simulink model "Impedance"  (R2022b)
settings: Solver=ode113  StartTime=0.0  StopTime=30  RelTol=1e-3
values from neighbouring files (symbols this model uses):
  a_1 = 1    [parameters.m]
  a_2 = 1    [parameters.m]
  kp_1 = 2500    [parameters.m]
  kp_2 = 2500    [parameters.m]
  md_1 = 100    [parameters.m]
  md_2 = 100    [parameters.m]
  xd_1 = 0.75    [parameters.m]
  xd_2 = 0.25    [parameters.m]
settings Model: Creator=eleves  LastModifiedBy=eleves
settings ModelReferenceCC: ModelReferenceMinAlgLoopOccurrences=on

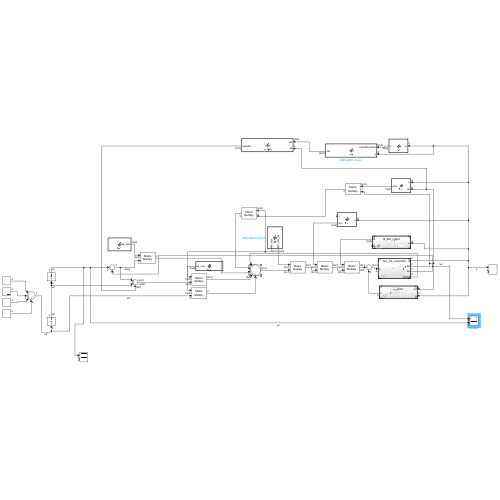
[thumbnail: Simulink's stored preview of the top-level diagram]
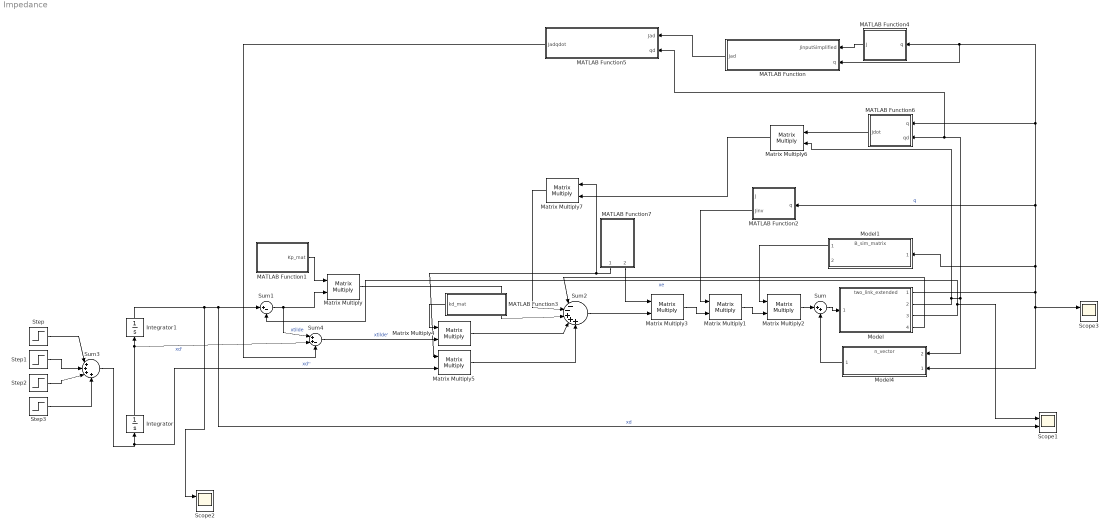
== system Impedance ==
  Integrator : Integrator  InitialCondition=[0;0]
  Integrator1 : Integrator  InitialCondition=[xd_1;xd_2]
  MATLAB Function : MATLAB Function  TreatAsAtomicUnit=on
  MATLAB Function1 : MATLAB Function  TreatAsAtomicUnit=on
  MATLAB Function2 : MATLAB Function  TreatAsAtomicUnit=on
  MATLAB Function3 : MATLAB Function  TreatAsAtomicUnit=on
  MATLAB Function4 : MATLAB Function  TreatAsAtomicUnit=on
  MATLAB Function5 : MATLAB Function  TreatAsAtomicUnit=on
  MATLAB Function6 : MATLAB Function  TreatAsAtomicUnit=on
  MATLAB Function7 : MATLAB Function  TreatAsAtomicUnit=on
  Matrix Multiply{,1..7} (8 alike) : Product  Multiplication=Matrix(*)
  Model : ModelReference  ModelNameDialog=two_link_extended.slx  SimulationMode=Normal  ModelReferenceVersion=1.3
  Model1 : ModelReference  ModelNameDialog=B_sim_matrix.slx  SimulationMode=Normal  ModelReferenceVersion=13.0
  Model4 : ModelReference  ModelNameDialog=n_vector.slx  SimulationMode=Normal  ModelReferenceVersion=1.3
      settings: PortSchema="{\"entries\":[{\"content\":{\"sides\":[{\"content\":{\"connectorIds\":[\"In2\",\"In1\"]},\"type\":\"ConnectorPlacement.EquallySpacedRectSide\",\"uuid\":\"0004a852-6b57-412e-a247-f7a948c02aef\"},{\"content\":{\"connectorIds\":[\"Out1\"],\"side\":\"RIGHT\"},\"type\":\"ConnectorPlacement.EquallySpacedRectSide\",\"uuid\":\"2c6a1f56-b264-4a50-8175-f4e8d5862eda\"},{\"content\":{\"connectorIds\":[],\"side\":\"TOP\"},\"type\":\"ConnectorPlacement.EquallySpacedRectSide\",\"uuid\":\"b3451316-5974-4a81-98c7-74555a3ec881\"}]},\"type\":\"ConnectorPlacement.EquallySpacedConnector\",\"uuid\":\"ac2390f0-df41-4187-a0e3-0c9a5394d303\"}],\"packageUris\":[\"http://schema.mathworks.com/mf0/Connector/R2020b\"],\"version\":\"1.0\"}"
  Scope1 : Scope  NumInputPorts=2
  Scope2 : Scope  NumInputPorts=2
  Scope3 : Scope  NumInputPorts=2
  Step : Step  Time=0  Before=[0.0;0.00]  After=[0.1;0.05]  SampleTime=0
  Step1 : Step  Before=[0.0;0.00]  After=[-0.1;-0.05]  SampleTime=0
  Step2 : Step  Time=5  Before=[0.0;0.00]  After=[-0.1;-0.05]  SampleTime=0
  Step3 : Step  Time=6  Before=[0.0;0.00]  After=[0.1;0.05]  SampleTime=0
  Sum : Sum  Inputs=|++
  Sum1 : Sum  Inputs=|+-
  Sum2 : Sum  Inputs=|--+++
  Sum3 : Sum  Inputs=|++++
  Sum4 : Sum  Inputs=|++-
  wires:
  Sum1/1 -> Sum4/1, Matrix Multiply/2  "xtilde"
  MATLAB Function1/1(Kp_mat) -> Matrix Multiply/1
  Model4/1 -> Sum/2
  Model1/1 -> Matrix Multiply2/1
  Matrix Multiply2/1 -> Sum/1
  Matrix Multiply1/1 -> Matrix Multiply2/2
  MATLAB Function2/2(Jinv) -> Matrix Multiply1/1
  Matrix Multiply3/1 -> Matrix Multiply1/2
  MATLAB Function7/2(Md_mat_inv) -> Matrix Multiply3/1
  Sum2/1 -> Matrix Multiply3/2
  Step/1 -> Sum3/1
  Step1/1 -> Sum3/2
  Step2/1 -> Sum3/3
  Step3/1 -> Sum3/4
  Sum3/1 -> Matrix Multiply5/2, Integrator/1  "xd''"
  Integrator1/1 -> Scope2/1, Scope1/2, Sum1/1  "xd"
  Matrix Multiply/1 -> Sum2/3
  Integrator/1 -> Integrator1/1, Sum4/2  "xd'"
  MATLAB Function3/1(kd_mat) -> Matrix Multiply4/1
  Sum4/1 -> Matrix Multiply4/2  "xtilde'"
  Matrix Multiply4/1 -> Sum2/4
  MATLAB Function7/1(Md_mat) -> Matrix Multiply7/1, Matrix Multiply5/1
  Matrix Multiply5/1 -> Sum2/5
  MATLAB Function6/1(Jdot) -> Matrix Multiply6/1
  Matrix Multiply6/1 -> Matrix Multiply7/2
  Matrix Multiply7/1 -> Sum2/2
  Model/1 -> Model1/1, MATLAB Function2/1(q), MATLAB Function/2(q), MATLAB Function4/1(q), MATLAB Function6/1(q), Scope3/1, Model4/1  "q"
  Sum/1 -> Model/1
  Model/2 -> Model4/2, MATLAB Function5/2(qd), MATLAB Function6/2(qd), Matrix Multiply6/2
  Model/3 -> Sum1/2, Scope1/1  "xe"
  Model/4 -> Sum2/1
  MATLAB Function4/1(J) -> MATLAB Function/1(JinputSimplified)
  MATLAB Function/1(Jad) -> MATLAB Function5/1(Jad)
  MATLAB Function5/1(Jadqdot) -> Sum4/3

== matlab function Impedance/MATLAB Function1 ==
  data: Kp_mat output; kp_1 parameter; kp_2 parameter
function Kp_mat = fcn(kp_1, kp_2)
    Kp_mat = [kp_1,0;
              0,kp_2];
end

== matlab function Impedance/MATLAB Function ==
  data: JinputSimplified input; Jad output; q input
function Jad = fcn(JinputSimplified,q)
    theta1 = q(1);
    theta2 = q(2);
    Ro3 = [ cos(theta1+theta2),-sin(theta1+theta2);
            sin(theta1+theta2),cos(theta1+theta2)];
    Ro3 = Ro3';
    Jad_temp = JinputSimplified(1:2,1:2);
    Jad_temp = Ro3*Jad_temp;
    Jad = Jad_temp;
end

== matlab function Impedance/MATLAB Function2 ==
  data: q input; J output; a_1 parameter; a_2 parameter; Jinv output
function [J,Jinv] = fcn(q,a_1, a_2)
    theta1 = q(1);
    theta2 = q(2);
    J = [-a_1*sin(theta1)-a_2*sin(theta1+theta2),-a_2*sin(theta1+theta2);
        a_1*cos(theta1)+a_2*cos(theta1+theta2),a_2*cos(theta1+theta2)];
    Jinv = pinv(J);

end

== matlab function Impedance/MATLAB Function3 ==
  data: kd_mat output; kp_1 parameter; kp_2 parameter
function kd_mat = fcn(kp_1, kp_2)
    kd_mat = [kp_1,0;
              0,kp_2];
end

== matlab function Impedance/MATLAB Function4 ==
  data: q input; J output; a_1 parameter; a_2 parameter
function J = fcn(q,a_1, a_2)
    theta1 = q(1);
    theta2 = q(2);
    J = [-a_1*sin(theta1)-a_2*sin(theta1+theta2),-a_2*sin(theta1+theta2),0;
        a_1*cos(theta1)+a_2*cos(theta1+theta2),a_2*cos(theta1+theta2),0;
        0,0,0;
        0,0,0;
        0,0,0;
        1,1,1;];

end

== matlab function Impedance/MATLAB Function5 ==
  data: Jad input; Jadqdot output; qd input
function Jadqdot = multiply(Jad,qd)
    qd = [qd(1);qd(2)];
    Jadqdot = Jad*qd;
end

== matlab function Impedance/MATLAB Function6 ==
  data: q input; qd input; Jdot output; a_1 parameter; a_2 parameter
function Jdot = fcn(q,qd,a_1, a_2)
    theta1 = q(1);
    theta2 = q(2);
    theta1d = qd(1);
    theta2d = qd(2);
    Jdot = [-a_1*theta1d*cos(theta1)-a_2*(theta1d+theta2d)*cos(theta1+theta2),-a_2*(theta1d+theta2d)*cos(theta1+theta2);
        -a_1*theta1d*sin(theta1)-a_2*(theta1d+theta2d)*sin(theta1+theta2),-a_2*(theta1d+theta2d)*sin(theta1+theta2)];

end

== matlab function Impedance/MATLAB Function7 ==
  data: Md_mat output; md_1 parameter; md_2 parameter; Md_mat_inv output
function [Md_mat,Md_mat_inv] = fcn(md_1, md_2)
    Md_mat = [md_1,0;
              0,md_2];
    Md_mat_inv = inv(Md_mat);
end
